simulink model "momentum_unload_test_simple"  (R2016b)
settings: Solver=VariableStepAuto  StartTime=0.0  StopTime=5400  MinStep=0.001  RelTol=1e-3
values from neighbouring files (symbols this model uses):
  fsw_params = init_fsw_params()    [momentum_unload_test_init.m]
undefined symbols (not defined in the file or in its folder): env_acc_eci, init_pos_eci, init_vel_eci, mag_vector_eci, sim_params
libraries: aerolibutil x2, bus_stubs_template x2, dynamics_lib x1, momentum_dump_lib_test x1, pd_control_lib x1, RW_assembly_simple_lib x1, command_processing x1, actuators_lib x1, tle2eci_coarse_lib x1
settings Model: Creator=taylorreynolds  LastModifiedBy=evich

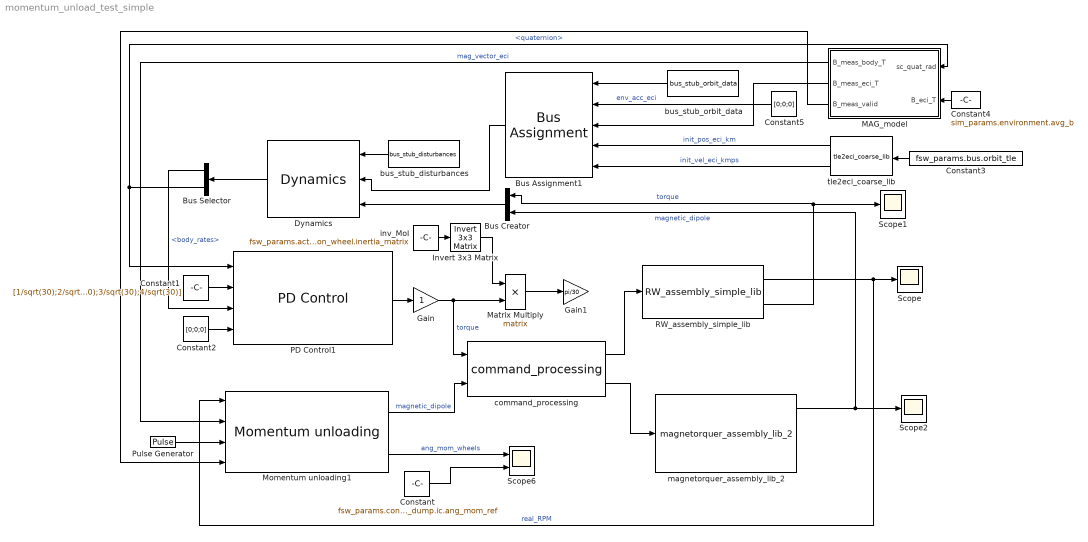
== system momentum_unload_test_simple ==
  Bus Assignment1 : BusAssignment  AssignedSignals=env_acc_eci,mag_vector_eci,init_pos_eci,init_vel_eci
  Bus Creator : BusCreator  Inputs=2
  Bus Selector : BusSelector  OutputSignals=body_rates,quaternion
  Constant : Constant  Value=fsw_params.control.p_dump.ic.ang_mom_ref
  Constant1 : Constant  Value=[1/sqrt(30);2/sqrt(30);3/sqrt(30);4/sqrt(30)]
  Constant2 : Constant  Value=[0;0;0]
  Constant3 : Constant  Value=fsw_params.bus.orbit_tle
  Constant4 : Constant  Value=sim_params.environment.avg_b
  Constant5 : Constant  Value=[0;0;0]
  Dynamics : dynamics_lib/Dynamics
  Gain : Gain
  Gain1 : Gain  Gain=pi/30
  Invert 3x3 Matrix : aerolibutil/Invert  3x3 Matrix
  MAG_model : Subsystem
  Matrix Multiply : Product  Multiplication=Matrix(*)
  Momentum unloading1 : momentum_dump_lib_test/Momentum unloading
  PD Control1 : pd_control_lib/PD Control
  Pulse Generator : DiscretePulseGenerator  PulseType=Time based  Period=fsw_params.actuators.ppt.sync_pulse  PulseWidth=fsw_params.actuators.ppt.t_charge_pct
  RW_assembly_simple_lib : RW_assembly_simple_lib/RW_assembly_simple_lib  natural_frequency=100  damping_ratio=1  max_rate=100000
  Scope : Scope
  Scope1 : Scope
  Scope2 : Scope
  Scope6 : Scope  NumInputPorts=2
  bus_stub_disturbances : bus_stubs_template/bus_stub_disturbances
  bus_stub_orbit_data : bus_stubs_template/bus_stub_orbit_data
  command_processing : command_processing/command_processing
  inv_MoI : Constant  Value=fsw_params.actuators.reaction_wheel.inertia_matrix
  magnetorquer_assembly_lib_2 : actuators_lib/Actuators/magnetorquer_assembly_lib_2
  tle2eci_coarse_lib : tle2eci_coarse_lib/tle2eci_coarse_lib
  wires:
  magnetorquer_assembly_lib_2/1 -> Bus Creator/2, Scope2/1  "magnetic_dipole"
  RW_assembly_simple_lib/2 -> Bus Creator/1, Scope1/1  "torque"
  RW_assembly_simple_lib/1 -> Momentum unloading1/1, Scope/1  "real_RPM"
  Momentum unloading1/1 -> command_processing/2  "magnetic_dipole"
  Pulse Generator/1 -> Momentum unloading1/3
  Momentum unloading1/2 -> Scope6/1  "ang_mom_wheels"
  Constant1/1 -> PD Control1/2
  Constant2/1 -> PD Control1/4
  Constant/1 -> Scope6/2
  PD Control1/1 -> Gain/1
  Gain/1 -> Matrix Multiply/2, command_processing/1  "torque"
  command_processing/2 -> magnetorquer_assembly_lib_2/1
  Dynamics/1 -> Bus Selector/1
  Bus Selector/2 -> MAG_model/1(sc_quat_rad), PD Control1/1  "<quaternion>"
  Bus Selector/1 -> PD Control1/3  "<body_rates>"
  Bus Creator/1 -> Dynamics/3
  MAG_model/3(B_meas_valid) -> Momentum unloading1/4
  Constant3/1 -> tle2eci_coarse_lib/1
  tle2eci_coarse_lib/1 -> Bus Assignment1/4  "init_pos_eci_km"
  tle2eci_coarse_lib/2 -> Bus Assignment1/5  "init_vel_eci_kmps"
  MAG_model/1(B_meas_body_T) -> Momentum unloading1/2  "mag_vector_eci"
  Constant4/1 -> MAG_model/2(B_eci_T)
  Constant5/1 -> Bus Assignment1/2  "env_acc_eci"
  bus_stub_disturbances/1 -> Dynamics/1
  bus_stub_orbit_data/1 -> Bus Assignment1/1
  Bus Assignment1/1 -> Dynamics/2
  MAG_model/2(B_meas_eci_T) -> Bus Assignment1/3
  Matrix Multiply/1 -> Gain1/1
  inv_MoI/1 -> Invert 3x3 Matrix/1
  Invert 3x3 Matrix/1 -> Matrix Multiply/1
  command_processing/1 -> RW_assembly_simple_lib/1

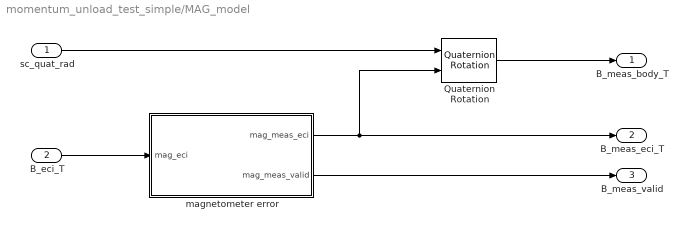
== system momentum_unload_test_simple/MAG_model ==
  sc_quat_rad : Inport
  B_eci_T : Inport  Port=2
  Quaternion Rotation : aerolibutil/Quaternion Rotation
  magnetometer error : Subsystem
  B_meas_body_T : Outport
  B_meas_eci_T : Outport  Port=2
  B_meas_valid : Outport  Port=3
  wires:
  sc_quat_rad/1 -> Quaternion Rotation/1
  B_eci_T/1 -> magnetometer error/1(mag_eci)
  magnetometer error/1(mag_meas_eci) -> Quaternion Rotation/2, B_meas_eci_T/1
  Quaternion Rotation/1 -> B_meas_body_T/1
  magnetometer error/2(mag_meas_valid) -> B_meas_valid/1

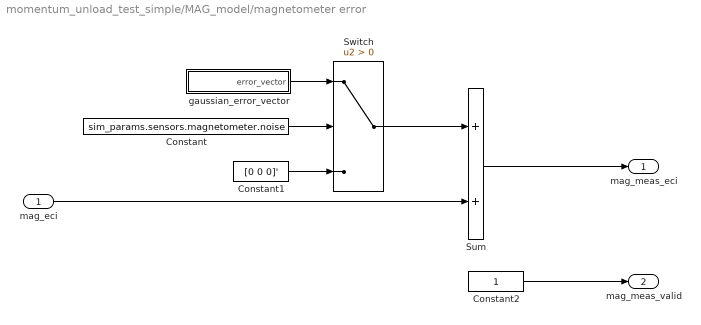
== system momentum_unload_test_simple/MAG_model/magnetometer error ==
  mag_eci : Inport
  Constant : Constant  Value=sim_params.sensors.magnetometer.noise
  Constant1 : Constant  Value=[0 0 0]'
  Constant2 : Constant
  Sum : Sum
  Switch : Switch  Criteria=u2 > Threshold
  gaussian_error_vector : Subsystem
  mag_meas_eci : Outport
  mag_meas_valid : Outport  Port=2
  wires:
  Constant2/1 -> mag_meas_valid/1
  Switch/1 -> Sum/1
  Constant1/1 -> Switch/3
  Constant/1 -> Switch/2
  gaussian_error_vector/1(error_vector) -> Switch/1
  Sum/1 -> mag_meas_eci/1
  mag_eci/1 -> Sum/2

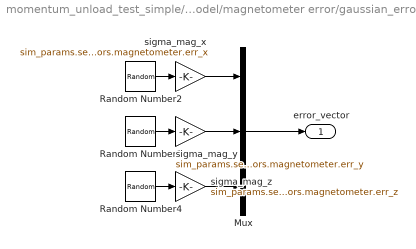
== system momentum_unload_test_simple/MAG_model/magnetometer error/gaussian_error_vector ==
  Mux : Mux  Inputs=3
  Random Number2 : RandomNumber  SampleTime=sim_params.sensors.magnetometer.sample_time_s
  Random Number3 : RandomNumber  Seed=1  SampleTime=sim_params.sensors.magnetometer.sample_time_s
  Random Number4 : RandomNumber  Seed=2  SampleTime=sim_params.sensors.magnetometer.sample_time_s
  sigma_mag_x : Gain  Gain=sim_params.sensors.magnetometer.err_x
  sigma_mag_y : Gain  Gain=sim_params.sensors.magnetometer.err_y
  sigma_mag_z : Gain  Gain=sim_params.sensors.magnetometer.err_z
  error_vector : Outport
  wires:
  Random Number2/1 -> sigma_mag_x/1
  Random Number4/1 -> sigma_mag_z/1
  Random Number3/1 -> sigma_mag_y/1
  sigma_mag_x/1 -> Mux/1
  sigma_mag_y/1 -> Mux/2
  Mux/1 -> error_vector/1
  sigma_mag_z/1 -> Mux/3
